simulink model "hexapod_with_floor"  (R2014b)
settings: Solver=ode23s  StartTime=0.0  StopTime=20  MaxStep=1e-2  RelTol=1e-5  AbsTol=1e-6
undefined symbols (not defined in the file): X, Y, Z
libraries: HexapodLib x8, sm_lib x5, nesl_utility x3, simulink_extras x2, simulink x2, fl_lib x1
settings Model: Creator=Sebastian  LastModifiedBy=Sebastian
settings SolverCC: SolverResetMethod=Robust
settings DiagnosticsConfigSet: SimMechanicsRigidlyBoundBlock=none

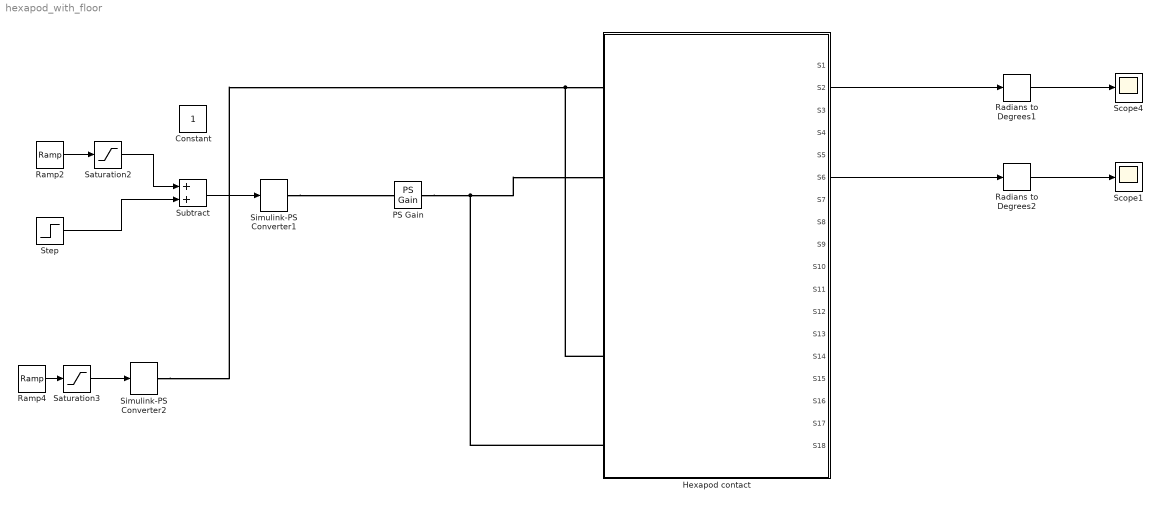
== system hexapod_with_floor ==
  Constant : Constant
  Hexapod contact : Subsystem  AncestorBlock=HexapodLib/Hexapod contact
  PS Gain : fl_lib/Physical Signals/Functions/PS Gain  gain=-1
  Radians to Degrees1 : simulink_extras/Transformations/Radians to Degrees
  Radians to Degrees2 : simulink_extras/Transformations/Radians to Degrees
  Ramp2 : simulink/Sources/Ramp  slope=-0.3  start=1  X0=0
  Ramp4 : simulink/Sources/Ramp  slope=0.15  start=15  X0=0
  Saturation2 : Saturate  UpperLimit=1.5  LowerLimit=-1.5
  Saturation3 : Saturate  UpperLimit=1.5  LowerLimit=-1.5
  Scope1 : Scope
      settings: ShowLegends=on  YMin=0  YMax=60  MaxDataPoints=50000
  Scope4 : Scope
      settings: ShowLegends=on  YMin=-20  YMax=180  MaxDataPoints=50000
  Simulink-PS Converter1 : nesl_utility/Simulink-PS Converter  PhysicalDomain=network_engine_domain  SubClassName=ps_input  LeftPortType=input  RightPortType=output  PseudoPeriodic=off  Frequencies=[]  NoiseDistribution=none  NoiseParameters=[]  Unit=N*m  AffineConversion=off  InputFiltering=on  SimscapeFilterOrder=2  InputFilterTimeConstant=0.001  UdotUserProvided=1
  Simulink-PS Converter2 : nesl_utility/Simulink-PS Converter  PhysicalDomain=network_engine_domain  SubClassName=ps_input  LeftPortType=input  RightPortType=output  PseudoPeriodic=off  Frequencies=[]  NoiseDistribution=none  NoiseParameters=[]  Unit=N*m  AffineConversion=off  InputFiltering=on  SimscapeFilterOrder=2  InputFilterTimeConstant=0.001  UdotUserProvided=1
  Step : Step  Time=30  After=0.7  SampleTime=0
  Subtract : Sum
  wires:
  Ramp2/1 -> Saturation2/1
  Saturation2/1 -> Subtract/1
  Subtract/1 -> Simulink-PS Converter1/1
  Step/1 -> Subtract/2
  Saturation3/1 -> Simulink-PS Converter2/1
  Radians to Degrees1/1 -> Scope4/1
  Radians to Degrees2/1 -> Scope1/1
  Hexapod contact/6(S6) -> Radians to Degrees2/1
  Hexapod contact/2(S2) -> Radians to Degrees1/1
  Ramp4/1 -> Saturation3/1
  connections:
  Simulink-PS Converter1/RConn1 -- PS Gain/LConn1
  PS Gain/RConn1 -- Hexapod contact/LConn18 -- Hexapod contact/LConn6
  Simulink-PS Converter2/RConn1 -- Hexapod contact/LConn14 -- Hexapod contact/LConn2

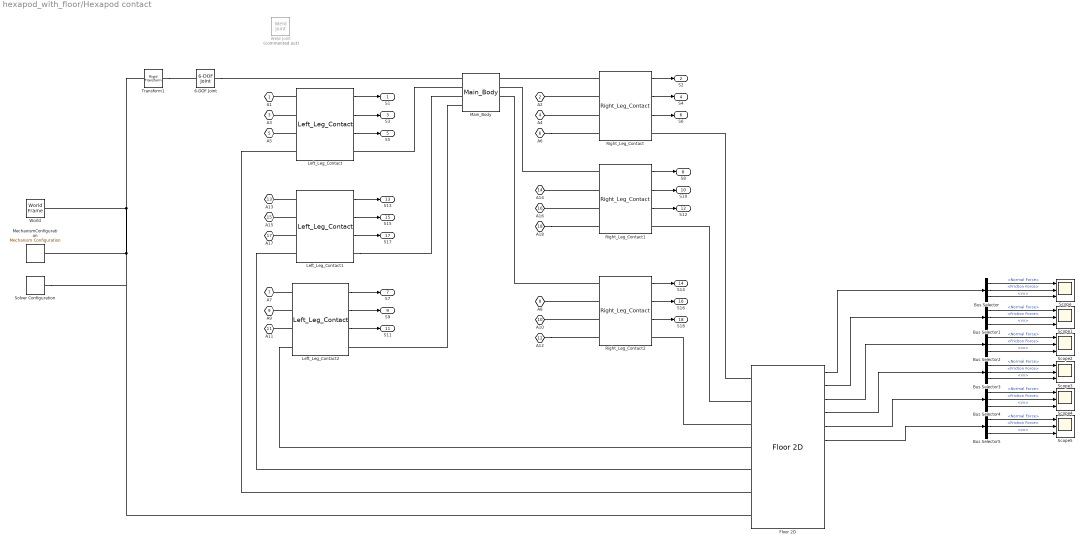
== system hexapod_with_floor/Hexapod contact ==
  6-DOF Joint : sm_lib/Joints/6-DOF Joint  SenseConstraintForce=off  SenseConstraintForceX=off  SenseConstraintForceY=off  SenseConstraintForceZ=off  SenseConstraintTorque=off  SenseConstraintTorqueX=off  SenseConstraintTorqueY=off  SenseConstraintTorqueZ=off  SenseTotalForce=off  SenseTotalForceX=off  SenseTotalForceY=off  SenseTotalForceZ=off  SenseTotalTorque=off  SenseTotalTorqueX=off  SenseTotalTorqueY=off  SenseTotalTorqueZ=off  CompositeWrenchDir=FollowerOnBase  CompositeWrenchFrame=BaseFrame  PxEquilibriumPosition=0  PxEquilibriumPositionUnits=m  PxSpringStiffness=0  PxSpringStiffnessUnits=N/m  PxDampingCoefficient=0  PxDampingCoefficientUnits=N/(m/s)  PxTorqueActuationMode=NoTorque  PxMotionActuationMode=ComputedMotion  PxSensePosition=off  PxSenseVelocity=off  PxSenseAcceleration=off  PxSenseTorqueForce=off  PxPositionTargetValue=0  PxPositionTargetValueUnits=m  PxPositionTargetSpecify=off  PxPositionTargetPriority=High  PxVelocityTargetValue=0  PxVelocityTargetValueUnits=m/s  PxVelocityTargetSpecify=off  PxVelocityTargetPriority=High  PyEquilibriumPosition=0  PyEquilibriumPositionUnits=m  PySpringStiffness=0  PySpringStiffnessUnits=N/m  PyDampingCoefficient=0  PyDampingCoefficientUnits=N/(m/s)  PyTorqueActuationMode=NoTorque  PyMotionActuationMode=ComputedMotion  PySensePosition=off  PySenseVelocity=off  PySenseAcceleration=off  PySenseTorqueForce=off  PyPositionTargetValue=0  PyPositionTargetValueUnits=m  PyPositionTargetSpecify=off  PyPositionTargetPriority=High  PyVelocityTargetValue=0  PyVelocityTargetValueUnits=m/s  PyVelocityTargetSpecify=off  PyVelocityTargetPriority=High  PzEquilibriumPosition=0  PzEquilibriumPositionUnits=m  PzSpringStiffness=0  PzSpringStiffnessUnits=N/m  PzDampingCoefficient=0  PzDampingCoefficientUnits=N/(m/s)  PzTorqueActuationMode=NoTorque  PzMotionActuationMode=ComputedMotion  PzSensePosition=off  PzSenseVelocity=off  PzSenseAcceleration=off  PzSenseTorqueForce=off  PzPositionTargetValue=0  PzPositionTargetValueUnits=m  PzPositionTargetSpecify=off  PzPositionTargetPriority=High  PzVelocityTargetValue=0  PzVelocityTargetValueUnits=m/s  PzVelocityTargetSpecify=off  PzVelocityTargetPriority=High  SphDefPosRotationMethod=None  SphDefPosRotationAngleUnits=deg  SphDefPosRotationStandardAxis=+Z  SphDefPosRotationAngle=0.0  SphDefPosRotationArbitraryAxis=[0 0 1]  SphDefPosFollAlignAxisA=+X  SphDefPosBaseAlignAxisA=+Y  SphDefPosFollAlignAxisB=+Y  SphDefPosBaseAlignAxisB=+Z  SphDefPosRotationMatrix=[1 0 0; 0 1 0; 0 0 1]  SphEqPosRotationMethod=None  SphEqPosRotationAngleUnits=deg  SphEqPosRotationStandardAxis=+Z  SphEqPosRotationAngle=0.0  SphEqPosRotationArbitraryAxis=[0 0 1]  SphEqPosFollAlignAxisA=+X  SphEqPosBaseAlignAxisA=+Y  SphEqPosFollAlignAxisB=+Y  SphEqPosBaseAlignAxisB=+Z  SphEqPosRotationMatrix=[1 0 0; 0 1 0; 0 0 1]  SphSpringStiffness=0  SphSpringStiffnessUnits=N*m/deg  SphDampingCoefficient=0  SphDampingCoefficientUnits=N*m/(deg/s)  SphActuateTorqueX=off  SphActuateTorqueY=off  SphActuateTorqueZ=off  SphActuateTorque=off  SphTorqueActuationMode=NoTorque  SphMotionActuationMode=ComputedMotion  SphActuationFrame=BaseFrame  SphSensePosition=off  SphSenseVelocityX=off  SphSenseVelocityY=off  SphSenseVelocityZ=off  SphSenseVelocity=off  SphSenseAccelerationX=off  SphSenseAccelerationY=off  SphSenseAccelerationZ=off  SphSenseAcceleration=off  SphSenseTorqueX=off  SphSenseTorqueY=off  SphSenseTorqueZ=off  SphSenseTorqueForce=off  SphSensingFrame=BaseFrame  SphPositionTargetRotationMethod=None  SphPositionTargetRotationAngleUnits=deg  SphPositionTargetRotationStandardAxis=+Z  SphPositionTargetRotationAngle=0.0  SphPositionTargetRotationArbitraryAxis=[0 0 1]  SphPositionTargetFollAlignAxisA=+X  SphPositionTargetBaseAlignAxisA=+Y  SphPositionTargetFollAlignAxisB=+Y  SphPositionTargetBaseAlignAxisB=+Z  SphPositionTargetRotationMatrix=[1 0 0; 0 1 0; 0 0 1]  SphPositionTargetSpecify=off  SphPositionTargetPriority=High  SphVelocityTargetValue=[0 0 0]  SphVelocityTargetValueUnits=deg/s  SphVelocityTargetSpecify=off  SphVelocityTargetPriority=High  SphVelocityTargetInFollowerFrame=on  BlockFunction=simmechanics.library.joints.sixdof_joint
  Bus Selector{,1..5} (6 alike) : BusSelector  OutputSignals=Normal Force,Friction Force,Frame Sep.vx
  Floor 2D : HexapodLib/Floor 2D  my_k=0.5  my_s=0.7  v_th=0.0001
  Left_Leg_Contact : HexapodLib/Left_Leg_Contact  SystemSampleTime=-1
  Left_Leg_Contact1 : HexapodLib/Left_Leg_Contact  SystemSampleTime=-1
  Left_Leg_Contact2 : HexapodLib/Left_Leg_Contact  SystemSampleTime=-1
  Main_Body : HexapodLib/Main_Body  SystemSampleTime=-1
  MechanismConfiguration : sm_lib/Utilities/Mechanism Configuration  UniformGravity=Constant  GravityVector=[0 0 -9.81]  GravityUnits=m/s^2  LinearizationDelta=0.001  BlockFunction=simmechanics.library.utilities.mechanism_configuration
  Right_Leg_Contact : HexapodLib/Right_Leg_Contact  SystemSampleTime=-1
  Right_Leg_Contact1 : HexapodLib/Right_Leg_Contact  SystemSampleTime=-1
  Right_Leg_Contact2 : HexapodLib/Right_Leg_Contact  SystemSampleTime=-1
  Scope{,1..5} (6 alike) : Scope  NumInputPorts=3
      Scope settings: YMin=0.5~2e-05~-1.1e-06  YMax=2~0.00011~-4e-07
      Scope1 settings: YMin=-5~-5~-5  YMax=5~5~5
      Scope2 settings: YMin=-5~-5~-5  YMax=5~5~5
      Scope3 settings: YMin=-5~-5~-5  YMax=5~5~5  SaveName=ScopeData2
      Scope4 settings: YMin=-5~-5~-5  YMax=5~5~5  SaveName=ScopeData3
      Scope5 settings: YMin=-5~-5~-5  YMax=5~5~5  SaveName=ScopeData4
  Solver Configuration : nesl_utility/Solver Configuration  PhysicalDomain=network_engine_domain  SubClassName=solver  LeftPortType=input  RightPortType=generic  Accelerate=off  Tones=[]  Harmonics=[]  SimulateNoise=off  Profile=off  UseLocalSampling=off  EnableSwitchedLinearOptims=on  FrequencyDomain=off  UseCCode=off  RelTol=0.001  AbsTol=1e-06  MinStep=1e-09  ToWorkspace=off  DoDC=off  ResidualTolerance=1e-09  UseLocalSolver=off  LocalSolverChoice=NE_BACKWARD_EULER_ADVANCER  LocalSolverSampleTime=0.001  DoFixedCost=off  MaxNonlinIter=3  MaxModeIter=2  LinearAlgebra=Sparse  DelaysMemoryBudget=1024  AutomaticFiltering=on  FilteringTimeConstant=0.001
  Transform1 : sm_lib/Frames and Transforms/Rigid Transform  TranslationMethod=Cartesian  TranslationLengthUnit=cm  TranslationStandardAxis=+Z  TranslationStandardOffset=0  TranslationCartesianOffset=[0 0 17]  TranslationROffset=0  TranslationROffsetUnits=m  TranslationZOffset=0  TranslationZOffsetUnits=m  TranslationThetaOffset=0  TranslationThetaOffsetUnits=deg  RotationMethod=None  RotationAngleUnits=rad  RotationStandardAxis=+Z  RotationAngle=0  RotationArbitraryAxis=[0 0 0]  FollAlignAxisA=+X  BaseAlignAxisA=+Y  FollAlignAxisB=+Y  BaseAlignAxisB=+Z  RotationMatrix=[1 0 0; 0 1 0; 0 0 1]  BlockFunction=simmechanics.library.frames_transforms.rigid_transform
  Weld Joint : sm_lib/Joints/Weld Joint  Commented=on  SenseConstraintForce=off  SenseConstraintForceX=off  SenseConstraintForceY=off  SenseConstraintForceZ=off  SenseConstraintTorque=off  SenseConstraintTorqueX=off  SenseConstraintTorqueY=off  SenseConstraintTorqueZ=off  SenseTotalForce=off  SenseTotalForceX=off  SenseTotalForceY=off  SenseTotalForceZ=off  SenseTotalTorque=off  SenseTotalTorqueX=off  SenseTotalTorqueY=off  SenseTotalTorqueZ=off  CompositeWrenchDir=FollowerOnBase  CompositeWrenchFrame=BaseFrame  BlockFunction=simmechanics.library.joints.weld_joint
  World : sm_lib/Frames and Transforms/World Frame  BlockFunction=simmechanics.library.frames_transforms.world_frame
  A1 : PMIOPort  Port=1  Side=Left
  A2 : PMIOPort  Port=2  Side=Left
  A3 : PMIOPort  Port=3  Side=Left
  A4 : PMIOPort  Port=4  Side=Left
  A5 : PMIOPort  Port=5  Side=Left
  A6 : PMIOPort  Port=6  Side=Left
  A7 : PMIOPort  Port=7  Side=Left
  A8 : PMIOPort  Port=8  Side=Left
  A9 : PMIOPort  Port=9  Side=Left
  A10 : PMIOPort  Port=10  Side=Left
  A11 : PMIOPort  Port=11  Side=Left
  A12 : PMIOPort  Port=12  Side=Left
  A13 : PMIOPort  Port=13  Side=Left
  A14 : PMIOPort  Port=14  Side=Left
  A15 : PMIOPort  Port=15  Side=Left
  A16 : PMIOPort  Port=16  Side=Left
  A17 : PMIOPort  Port=17  Side=Left
  A18 : PMIOPort  Port=18  Side=Left
  S1 : Outport
  S2 : Outport  Port=2
  S3 : Outport  Port=3
  S4 : Outport  Port=4
  S5 : Outport  Port=5
  S6 : Outport  Port=6
  S7 : Outport  Port=7
  S8 : Outport  Port=8
  S9 : Outport  Port=9
  S10 : Outport  Port=10
  S11 : Outport  Port=11
  S12 : Outport  Port=12
  S13 : Outport  Port=13
  S14 : Outport  Port=14
  S15 : Outport  Port=15
  S16 : Outport  Port=16
  S17 : Outport  Port=17
  S18 : Outport  Port=18
  wires:
  Floor 2D/6 -> Bus Selector5/1
  Floor 2D/5 -> Bus Selector4/1
  Floor 2D/4 -> Bus Selector3/1
  Floor 2D/3 -> Bus Selector2/1
  Floor 2D/2 -> Bus Selector1/1
  Floor 2D/1 -> Bus Selector/1
  Left_Leg_Contact/1 -> S1/1
  Left_Leg_Contact/2 -> S3/1
  Left_Leg_Contact/3 -> S5/1
  Left_Leg_Contact1/1 -> S13/1
  Left_Leg_Contact1/2 -> S15/1
  Left_Leg_Contact1/3 -> S17/1
  Left_Leg_Contact2/1 -> S7/1
  Left_Leg_Contact2/2 -> S9/1
  Left_Leg_Contact2/3 -> S11/1
  Right_Leg_Contact/1 -> S2/1
  Right_Leg_Contact/2 -> S4/1
  Right_Leg_Contact/3 -> S6/1
  Right_Leg_Contact1/1 -> S8/1
  Right_Leg_Contact1/2 -> S10/1
  Right_Leg_Contact1/3 -> S12/1
  Right_Leg_Contact2/1 -> S14/1
  Right_Leg_Contact2/2 -> S16/1
  Right_Leg_Contact2/3 -> S18/1
  Bus Selector/1 -> Scope/1  "<Normal Force>"
  Bus Selector/2 -> Scope/2  "<Friction Force>"
  Bus Selector/3 -> Scope/3  "<vx>"
  Bus Selector1/1 -> Scope1/1  "<Normal Force>"
  Bus Selector1/2 -> Scope1/2  "<Friction Force>"
  Bus Selector1/3 -> Scope1/3  "<vx>"
  Bus Selector2/1 -> Scope2/1  "<Normal Force>"
  Bus Selector2/2 -> Scope2/2  "<Friction Force>"
  Bus Selector2/3 -> Scope2/3  "<vx>"
  Bus Selector3/1 -> Scope3/1  "<Normal Force>"
  Bus Selector3/2 -> Scope3/2  "<Friction Force>"
  Bus Selector3/3 -> Scope3/3  "<vx>"
  Bus Selector4/1 -> Scope4/1  "<Normal Force>"
  Bus Selector4/2 -> Scope4/2  "<Friction Force>"
  Bus Selector4/3 -> Scope4/3  "<vx>"
  Bus Selector5/1 -> Scope5/1  "<Normal Force>"
  Bus Selector5/2 -> Scope5/2  "<Friction Force>"
  Bus Selector5/3 -> Scope5/3  "<vx>"
  connections:
  6-DOF Joint/RConn1 -- Main_Body/LConn1
  Floor 2D/LConn3 -- Right_Leg_Contact2/RConn1
  Floor 2D/LConn2 -- Right_Leg_Contact1/RConn1
  Floor 2D/LConn1 -- Right_Leg_Contact/RConn1
  Right_Leg_Contact1/LConn3 -- A16/RConn1
  Right_Leg_Contact1/LConn2 -- A14/RConn1
  Right_Leg_Contact2/LConn3 -- A10/RConn1
  Right_Leg_Contact2/LConn2 -- A8/RConn1
  Right_Leg_Contact2/LConn1 -- Main_Body/RConn3
  Right_Leg_Contact/LConn1 -- Main_Body/RConn1
  Transform1/LConn1 -- World/RConn1 -- MechanismConfiguration/RConn1 -- Solver Configuration/RConn1 -- Floor 2D/LConn7
  Left_Leg_Contact/LConn2 -- A3/RConn1
  Left_Leg_Contact/LConn1 -- A1/RConn1
  Right_Leg_Contact/LConn2 -- A2/RConn1
  Right_Leg_Contact1/LConn1 -- Main_Body/RConn2
  Right_Leg_Contact/LConn3 -- A4/RConn1
  Left_Leg_Contact2/LConn1 -- A7/RConn1
  Left_Leg_Contact2/LConn2 -- A9/RConn1
  Left_Leg_Contact1/LConn1 -- A13/RConn1
  Left_Leg_Contact1/LConn2 -- A15/RConn1
  Transform1/RConn1 -- 6-DOF Joint/LConn1
  A12/RConn1 -- Right_Leg_Contact2/LConn4
  A18/RConn1 -- Right_Leg_Contact1/LConn4
  A6/RConn1 -- Right_Leg_Contact/LConn4
  Left_Leg_Contact/LConn3 -- A5/RConn1
  Left_Leg_Contact1/LConn3 -- A17/RConn1
  Left_Leg_Contact2/LConn3 -- A11/RConn1
  Main_Body/LConn2 -- Left_Leg_Contact/RConn1
  Floor 2D/LConn6 -- Left_Leg_Contact/LConn4
  Left_Leg_Contact1/RConn1 -- Main_Body/LConn3
  Floor 2D/LConn5 -- Left_Leg_Contact1/LConn4
  Main_Body/LConn4 -- Left_Leg_Contact2/RConn1
  Floor 2D/LConn4 -- Left_Leg_Contact2/LConn4
